simulink model "BlakesSimulinkCode"  (R2019a)
settings: Solver=FixedStepAuto  StartTime=0.0  StopTime=10.0  RelTol=1e-3  EnableMultiTasking=on
libraries: vexarmcortexlib x15
settings Model: ExtModeTrigDuration=25  Creator=Blake Davis  LastModifiedBy=Blake Davis
settings OptimizationCC: EnhancedBackFolding=on  PassReuseOutputArgsAs=Individual arguments  MaxStackSize=64  OptimizeBlockOrder=speed  DifferentSizesBufferReuse=on  OptimizationCustomize=off
settings DebuggingCC: ParameterTunabilityLossMsg=error
settings HardwareCC: ProdBitPerPointer=32  ProdBitPerSizeT=32  ProdBitPerPtrDiffT=32  ProdLargestAtomicInteger=Long  ProdLargestAtomicFloat=Double  ProdWordSize=32  ProdHWDeviceType=ARM Compatible->ARM Cortex
settings SFSimCC: MATLABDynamicMemAlloc=off
settings RTWCC: SystemTargetFile=ert.tlc  HardwareBoard=ARM Cortex-based VEX Microcontroller  TLCOptions="-aInlineSetEventsForThisBaseRateFcn=TLC_FALSE -aSuppressMultiTaskScheduler=TLC_FALSE  -aRateBasedStepFcn=0"  TemplateMakefile=ert_default_tmf  GenerateReport=on  Toolchain=GNU Tools for VEX ARM Cortex  IncludeHyperlinkInReport=on  LaunchReport=on  GenerateTraceInfo=on  GenerateTraceReport=on  GenerateTraceReportSl=on  GenerateTraceReportSf=on  GenerateTraceReportEml=on
settings CodeAppCC: ForceParamTrailComments=on  IgnoreCustomStorageClasses=off  OperatorAnnotations=on  SimulinkDataObjDesc=on  SFDataObjDesc=on  InsertBlockDesc=on

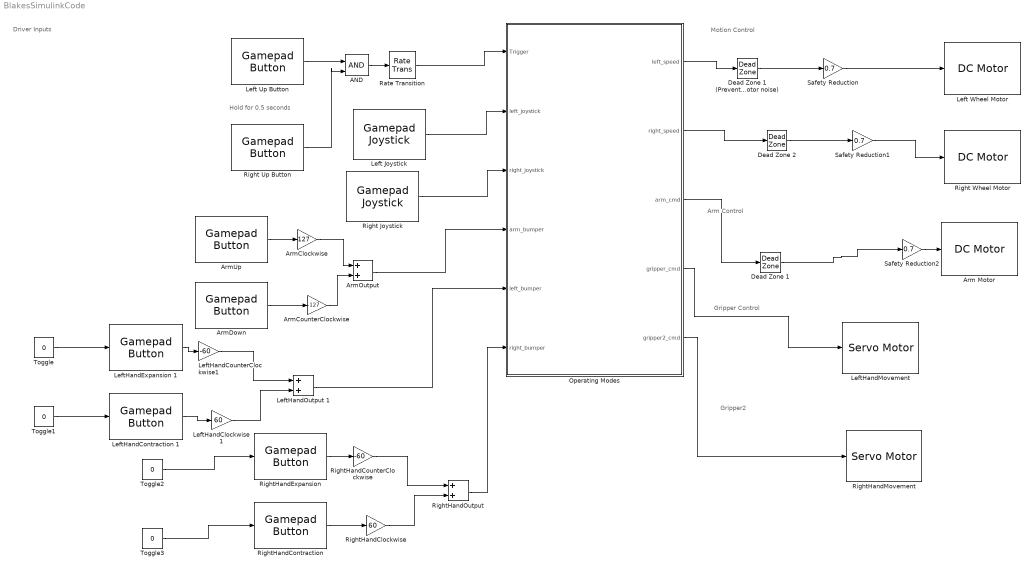
== system BlakesSimulinkCode ==
  note: Gripper Control
  note: Hold for 0.5 seconds
  note: Driver Inputs
  note: Motion Control
  note: Gripper2
  note: Arm Control
  AND : Logic  IconShape=distinctive  AllPortsSameDT=off  OutDataTypeStr=boolean
  Arm Motor : vexarmcortexlib/Actuators/DC Motor  motor=4  scaleFactor=1/13.5  SimulationOut=off
      settings: SourceProductName=Simulink Coder Support Package for ARM Cortex-based VEX Microcontroller  SourceProductBaseCode=EC_VEX_MICRO
  ArmClockwise : Gain  Gain=127
  ArmCounterClockwise : Gain  Gain=-127
  "ArmDown " : vexarmcortexlib/Gamepad/Gamepad Button  joystick=1  chan=7  button56=Up  button78=Down  SimulationIn=off  SampleTime=0.02
      settings: SourceProductName=Simulink Coder Support Package for ARM Cortex-based VEX Microcontroller  SourceProductBaseCode=EC_VEX_MICRO
  ArmOutput : Sum
  "ArmUp " : vexarmcortexlib/Gamepad/Gamepad Button  joystick=1  chan=7  button56=Up  button78=Up  SimulationIn=off  SampleTime=0.02
      settings: SourceProductName=Simulink Coder Support Package for ARM Cortex-based VEX Microcontroller  SourceProductBaseCode=EC_VEX_MICRO
  Dead Zone 1 : DeadZone  LowerValue=-30  UpperValue=30  SaturateOnIntegerOverflow=on
  Dead Zone 1 (Prevents motor noise) : DeadZone  LowerValue=-30  UpperValue=30  SaturateOnIntegerOverflow=on
  Dead Zone 2 : DeadZone  LowerValue=-30  UpperValue=30  SaturateOnIntegerOverflow=on
  Left Joystick : vexarmcortexlib/Gamepad/Gamepad Joystick  joystick=1  chan=3  SimulationIn=off  SampleTime=0.02
      settings: SourceProductName=Simulink Coder Support Package for ARM Cortex-based VEX Microcontroller  SourceProductBaseCode=EC_VEX_MICRO
  Left Up Button : vexarmcortexlib/Gamepad/Gamepad Button  joystick=1  chan=5  button56=Up  button78=Up  SimulationIn=off  SampleTime=0.5
      settings: SourceProductName=Simulink Coder Support Package for ARM Cortex-based VEX Microcontroller  SourceProductBaseCode=EC_VEX_MICRO
  Left Wheel Motor : vexarmcortexlib/Actuators/DC Motor  motor=9  scaleFactor=1/13.5  SimulationOut=off
      settings: SourceProductName=Simulink Coder Support Package for ARM Cortex-based VEX Microcontroller  SourceProductBaseCode=EC_VEX_MICRO
  LeftHandClockwise 1 : Gain  Gain=60
  LeftHandContraction 1 : vexarmcortexlib/Gamepad/Gamepad Button  joystick=1  chan=7  button56=Up  button78=Left  SimulationIn=on  SampleTime=0.02
      settings: SourceProductName=Simulink Coder Support Package for ARM Cortex-based VEX Microcontroller  SourceProductBaseCode=EC_VEX_MICRO
  LeftHandCounterClockwise1 : Gain  Gain=-60
  LeftHandExpansion 1 : vexarmcortexlib/Gamepad/Gamepad Button  joystick=1  chan=7  button56=Up  button78=Right  SimulationIn=on  SampleTime=0.02
      settings: SourceProductName=Simulink Coder Support Package for ARM Cortex-based VEX Microcontroller  SourceProductBaseCode=EC_VEX_MICRO
  LeftHandMovement : vexarmcortexlib/Actuators/Servo Motor  motor=5  scaleFactor=60/127  SimulationOut=off
      settings: SourceProductName=Simulink Coder Support Package for ARM Cortex-based VEX Microcontroller  SourceProductBaseCode=EC_VEX_MICRO
  LeftHandOutput 1 : Sum
  Operating Modes : Stateflow chart  TreatAsAtomicUnit=on
  Rate Transition : RateTransition
  Right Joystick : vexarmcortexlib/Gamepad/Gamepad Joystick  joystick=1  chan=2  SimulationIn=off  SampleTime=0.02
      settings: SourceProductName=Simulink Coder Support Package for ARM Cortex-based VEX Microcontroller  SourceProductBaseCode=EC_VEX_MICRO
  Right Up Button : vexarmcortexlib/Gamepad/Gamepad Button  joystick=1  chan=5  button56=Down  button78=Up  SimulationIn=off  SampleTime=0.5
      settings: SourceProductName=Simulink Coder Support Package for ARM Cortex-based VEX Microcontroller  SourceProductBaseCode=EC_VEX_MICRO
  Right Wheel Motor : vexarmcortexlib/Actuators/DC Motor  motor=2  scaleFactor=1/13.5  SimulationOut=off
      settings: SourceProductName=Simulink Coder Support Package for ARM Cortex-based VEX Microcontroller  SourceProductBaseCode=EC_VEX_MICRO
  "RightHandClockwise " : Gain  Gain=60
  "RightHandContraction " : vexarmcortexlib/Gamepad/Gamepad Button  joystick=1  chan=8  button56=Up  button78=Right  SimulationIn=on  SampleTime=0.02
      settings: SourceProductName=Simulink Coder Support Package for ARM Cortex-based VEX Microcontroller  SourceProductBaseCode=EC_VEX_MICRO
  RightHandCounterClockwise : Gain  Gain=-60
  "RightHandExpansion " : vexarmcortexlib/Gamepad/Gamepad Button  joystick=1  chan=8  button56=Up  button78=Left  SimulationIn=on  SampleTime=0.02
      settings: SourceProductName=Simulink Coder Support Package for ARM Cortex-based VEX Microcontroller  SourceProductBaseCode=EC_VEX_MICRO
  RightHandMovement : vexarmcortexlib/Actuators/Servo Motor  motor=6  scaleFactor=60/127  SimulationOut=off
      settings: SourceProductName=Simulink Coder Support Package for ARM Cortex-based VEX Microcontroller  SourceProductBaseCode=EC_VEX_MICRO
  "RightHandOutput " : Sum
  Safety Reduction : Gain  Gain=0.7
  Safety Reduction1 : Gain  Gain=0.7
  Safety Reduction2 : Gain  Gain=0.7
  Toggle{,1..3} (4 alike) : Constant  Value=0
      settings: OpenFcn=|
      | if strcmp('0',get_param(gcb, 'Value'))                        set_param(gcb, 'Value', '1');
      | else
      |             set_param(gcb, 'Value', '0');
      | end
  wires:
  Dead Zone 1/1 -> Safety Reduction2/1
  Operating Modes/3(arm_cmd) -> Dead Zone 1/1
  Safety Reduction2/1 -> Arm Motor/1
  LeftHandContraction 1/1 -> LeftHandClockwise 1/1
  LeftHandCounterClockwise1/1 -> LeftHandOutput 1/1
  LeftHandExpansion 1/1 -> LeftHandCounterClockwise1/1
  LeftHandClockwise 1/1 -> LeftHandOutput 1/2
  Toggle3/1 -> "RightHandContraction "/1
  Operating Modes/4(gripper_cmd) -> LeftHandMovement/1
  LeftHandOutput 1/1 -> Operating Modes/5(left_bumper)
  ArmOutput/1 -> Operating Modes/4(arm_bumper)
  Toggle/1 -> LeftHandExpansion 1/1
  Dead Zone 2/1 -> Safety Reduction1/1
  Operating Modes/2(right_speed) -> Dead Zone 2/1
  ArmClockwise/1 -> ArmOutput/1
  Left Up Button/1 -> AND/1
  ArmCounterClockwise/1 -> ArmOutput/2
  Toggle2/1 -> "RightHandExpansion "/1
  Rate Transition/1 -> Operating Modes/1(Trigger)
  Safety Reduction1/1 -> Right Wheel Motor/1
  "RightHandClockwise "/1 -> "RightHandOutput "/2
  Dead Zone 1 (Prevents motor noise)/1 -> Safety Reduction/1
  "ArmDown "/1 -> ArmCounterClockwise/1
  Operating Modes/5(gripper2_cmd) -> RightHandMovement/1
  "RightHandExpansion "/1 -> RightHandCounterClockwise/1
  Right Up Button/1 -> AND/2
  "RightHandContraction "/1 -> "RightHandClockwise "/1
  RightHandCounterClockwise/1 -> "RightHandOutput "/1
  Operating Modes/1(left_speed) -> Dead Zone 1 (Prevents motor noise)/1
  Left Joystick/1 -> Operating Modes/2(left_joystick)
  "RightHandOutput "/1 -> Operating Modes/6(right_bumper)
  Right Joystick/1 -> Operating Modes/3(right_joystick)
  AND/1 -> Rate Transition/1
  Toggle1/1 -> LeftHandContraction 1/1
  "ArmUp "/1 -> ArmClockwise/1
  Safety Reduction/1 -> Left Wheel Motor/1

== stateflow chart BlakesSimulinkCode/Operating Modes ==
  state DriverControl
    left_speed = left_joystick;
    right_speed = right_joystick;
    arm_cmd = arm_bumper;
    gripper_cmd = left_bumper;
    gripper2_cmd = right_bumper;
  state AutonomousMode
    state MoveForward
      en:
      right_speed = 100;
      left_speed = 100;
    state Grab
      en:
      gripper_cmd = 60;
      gripper2_cmd = 60;
    state TurnAround
      en:
      right_speed = 90;
      left_speed = -90;
    state MoveBackward
      en:
      right_speed = 100;
      left_speed = 100;
    state Stop
      en:
      right_speed = 0;
      left_speed = 0;
      Done = true;
    (default) -> MoveForward : {Done = false;
        | gripper_cmd = 0;
        | arm_cmd = 0;}
    MoveForward -> Grab : after(7,sec)
    Grab -> TurnAround : after(2,sec)
    TurnAround -> MoveBackward : after(4,sec)
    MoveBackward -> Stop : after(7,sec)
  (default) -> DriverControl
  DriverControl -> AutonomousMode : [Trigger]
  AutonomousMode -> DriverControl : [Trigger || Done]
  data: Trigger input; left_joystick input; right_joystick input; arm_bumper input; left_bumper input; right_bumper input; left_speed output; right_speed output; arm_cmd output; gripper_cmd output; Done local boolean; gripper2_cmd output
